simulink model "pwm dc motor"  (R2021a)
settings: Solver=VariableStepAuto  StartTime=0.0  StopTime=20  RelTol=1e-3
undefined symbols (not defined in the file or in its folder): sigbuilder_block
settings Model: Creator=hritw  LastModifiedBy=hritw

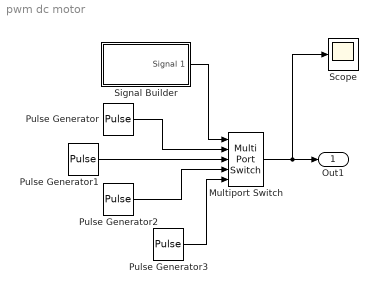
== system pwm dc motor ==
  Multiport Switch : MultiPortSwitch  Inputs=4
  Pulse Generator : DiscretePulseGenerator  PulseType=Time based  Amplitude=10  Period=10  PulseWidth=59.58
  Pulse Generator1 : DiscretePulseGenerator  PulseType=Time based  Amplitude=-10  Period=10  PulseWidth=5
  Pulse Generator2 : DiscretePulseGenerator  PulseType=Time based  Amplitude=4  Period=10  PulseWidth=5
  Pulse Generator3 : DiscretePulseGenerator  PulseType=Time based  Amplitude=16  Period=10  PulseWidth=5
  Scope : Scope
  Signal Builder : Subsystem  Tag=STV Subsys  LoadFcn=sigbuilder_block('load');  StartFcn=sigbuilder_block('start');  StopFcn=sigbuilder_block('stop');  ClipboardFcn=sigbuilder_block('clipboard');  mask(Sigbuilder block){tuvar=[0:10]}
      mask help: Simulink:masks:SigbuilderBlock_MD
      mask init:
      | if ~strcmp(get_param(bdroot(gcbh),'SimulationStatus'),'stopped') tuvar = sigbuilder_block('maskInit'); end
      settings: CopyFcn=sigbuilder_block('copy');  DeleteFcn=sigbuilder_block('delete');  ModelCloseFcn=sigbuilder_block('modelClose');  PreSaveFcn=sigbuilder_block('preSave');  PauseFcn=sigbuilder_block('pause');  ContinueFcn=sigbuilder_block('continue');  NameChangeFcn=sigbuilder_block('namechange');  OpenFcn=sigbuilder_block('open',[5.4 30 1141.2 522.6 ]);  CloseFcn=sigbuilder_block('close');
      mask Display: plot(0, 0, 100, 100,[2, 2, 32, 32, 2], [68, 8, 8, 68, 68],[32, 2], [38, 38], [32, 19, 2],[53, 60, 44], [32, 17, 17, 2],[16, 16, 31, 31]);txt = getActiveGroup(gcbh);text(2, 100, txt,'verticalAlignment', 'top');
  Out1 : Outport
  wires:
  Signal Builder/1(Signal 1) -> Multiport Switch/1
  Pulse Generator/1 -> Multiport Switch/2
  Pulse Generator1/1 -> Multiport Switch/3
  Pulse Generator2/1 -> Multiport Switch/4
  Pulse Generator3/1 -> Multiport Switch/5
  Multiport Switch/1 -> Scope/1, Out1/1

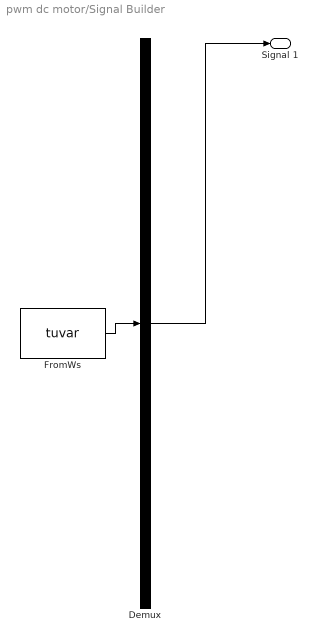
== system pwm dc motor/Signal Builder ==
  Demux : Demux  Tag=STV Demux  Outputs=1
      settings: DisplayOption=none
  FromWs : FromWorkspace  Tag=STV FromWs  VariableName=tuvar
      SigBuilderData=|
      | common.afterFinalStr = 'Extrapolate'
      | common.sampleTime = 0
      | dataSet.timeRange = [0 20]
      | dataSet.name = 'Group 1'
      | sbobj.Groups.Name = 'Group 1'
      | sbobj.Groups.Signals.Name = 'Signal 1'
      | sbobj.Groups.Signals.XData = [0 0.5 1 1.5 2 2.5 3 3 3.5 4 4.5 5 5.5 6 6 7 7.5 8 8.5 9 9.5 10 10 20]
      | sbobj.Groups.Signals.YData = [1 1 1 1 1 1 1 2 2 2 2 2 2 2 3 3 3 3 3 3 3 3 4 4]
      | sbobj.Groups.TimeRange = [0 20]
  Signal 1 : Outport  Tag=STV Outport
  wires:
  Demux/1 -> Signal 1/1
  FromWs/1 -> Demux/1
